simulink model "Quadrotor_eliminated_v2"  (R2020a)
settings: Solver=FixedStepAuto  StartTime=0.0  StopTime=options.T_train  FixedStep=options.dt  RelTol=1e-6
undefined symbols (not defined in the file or in its folder): options, Quad
libraries: neural x179, simulink x2
(part 3 of 10)

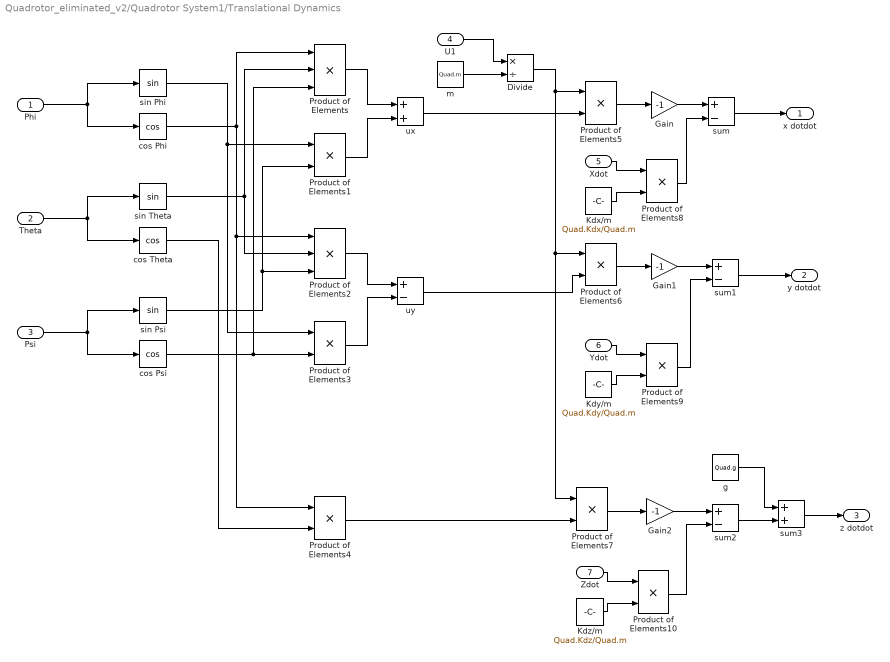
== system Quadrotor_eliminated_v2/Quadrotor System1/Translational Dynamics ==
  Phi : Inport
  Theta : Inport  Port=2
  Psi : Inport  Port=3
  U1 : Inport  Port=4
  Xdot : Inport  Port=5
  Ydot : Inport  Port=6
  Zdot : Inport  Port=7
  Divide : Product  Inputs=*/
  Gain : Gain  Gain=-1
  Gain1 : Gain  Gain=-1
  Gain2 : Gain  Gain=-1
  Kdx/m : Constant  Value=Quad.Kdx/Quad.m
  Kdy/m : Constant  Value=Quad.Kdy/Quad.m
  Kdz/m : Constant  Value=Quad.Kdz/Quad.m
  Product of Elements : Product  Inputs=3
  Product of Elements{1,3..10} (9 alike) : Product
  Product of Elements2 : Product  Inputs=3
  cos Phi : Trigonometry  Operator=cos
  cos Psi : Trigonometry  Operator=cos
  cos Theta : Trigonometry  Operator=cos
  g : Constant  Value=Quad.g
  m : Constant  Value=Quad.m
  sin Phi : Trigonometry
  sin Psi : Trigonometry
  sin Theta : Trigonometry
  sum : Sum  Inputs=+-
  sum1 : Sum  Inputs=+-
  sum2 : Sum  Inputs=+-
  sum3 : Sum
  ux : Sum
  uy : Sum  Inputs=+-
  x dotdot : Outport  VectorParamsAs1DForOutWhenUnconnected=off
  y dotdot : Outport  Port=2  VectorParamsAs1DForOutWhenUnconnected=off
  z dotdot : Outport  Port=3  VectorParamsAs1DForOutWhenUnconnected=off
  wires:
  Phi/1 -> sin Phi/1, cos Phi/1
  Theta/1 -> sin Theta/1, cos Theta/1
  Psi/1 -> sin Psi/1, cos Psi/1
  sin Theta/1 -> Product of Elements/2, Product of Elements2/2
  cos Psi/1 -> Product of Elements/3, Product of Elements3/2
  cos Phi/1 -> Product of Elements/1, Product of Elements2/1, Product of Elements4/1
  sin Phi/1 -> Product of Elements1/1, Product of Elements3/1
  sin Psi/1 -> Product of Elements1/2, Product of Elements2/3
  Product of Elements/1 -> ux/1
  Product of Elements1/1 -> ux/2
  ux/1 -> Product of Elements5/2
  Product of Elements2/1 -> uy/1
  Product of Elements3/1 -> uy/2
  uy/1 -> Product of Elements6/2
  cos Theta/1 -> Product of Elements4/2
  Product of Elements4/1 -> Product of Elements7/2
  U1/1 -> Divide/1
  m/1 -> Divide/2
  Divide/1 -> Product of Elements5/1, Product of Elements6/1, Product of Elements7/1
  sum3/1 -> z dotdot/1
  Product of Elements5/1 -> Gain/1
  Product of Elements6/1 -> Gain1/1
  Xdot/1 -> Product of Elements8/1
  Kdx/m/1 -> Product of Elements8/2
  Gain/1 -> sum/1
  Product of Elements8/1 -> sum/2
  sum/1 -> x dotdot/1
  Ydot/1 -> Product of Elements9/1
  Kdy/m/1 -> Product of Elements9/2
  Gain1/1 -> sum1/1
  Product of Elements9/1 -> sum1/2
  sum1/1 -> y dotdot/1
  Zdot/1 -> Product of Elements10/1
  Kdz/m/1 -> Product of Elements10/2
  Product of Elements7/1 -> Gain2/1
  g/1 -> sum3/1
  sum2/1 -> sum3/2
  Product of Elements10/1 -> sum2/2
  Gain2/1 -> sum2/1

== system Quadrotor_eliminated_v2/Quadrotor System2/Angular Velocities Transformation ==
  Theta : Inport
  Phi : Inport  Port=2
  Phi dot : Inport  Port=3
  Theta dot : Inport  Port=4
  Psi dot : Inport  Port=5
  Product : Product  RndMeth=Zero
  Product1 : Product  RndMeth=Zero
  Product2 : Product  Inputs=3  RndMeth=Zero
  Product3 : Product  RndMeth=Zero
  Product4 : Product  Inputs=3  RndMeth=Zero
  Sum : Sum  Inputs=+-
  Sum1 : Sum
  Sum2 : Sum
  sin : Trigonometry
  sin{1,4..6} (4 alike) : Trigonometry  Operator=cos
  sin2 : Trigonometry
  sin3 : Trigonometry
  p : Outport  VectorParamsAs1DForOutWhenUnconnected=off
  q : Outport  Port=2  VectorParamsAs1DForOutWhenUnconnected=off
  r : Outport  Port=3  VectorParamsAs1DForOutWhenUnconnected=off
  wires:
  Phi dot/1 -> Sum/1
  Theta/1 -> sin4/1, sin6/1, sin/1
  sin/1 -> Product/1
  Psi dot/1 -> Product/2, Product2/3, Product4/1
  Product/1 -> Sum/2
  Sum/1 -> p/1
  Phi/1 -> sin1/1, sin2/1, sin3/1, sin5/1
  sin1/1 -> Product1/1
  Theta dot/1 -> Product1/2, Product3/1
  Product1/1 -> Sum1/1
  sin2/1 -> Product2/1
  sin4/1 -> Product2/2
  Product2/1 -> Sum1/2
  Sum1/1 -> q/1
  sin3/1 -> Product3/2
  sin5/1 -> Product4/2
  sin6/1 -> Product4/3
  Product3/1 -> Sum2/1
  Product4/1 -> Sum2/2
  Sum2/1 -> r/1

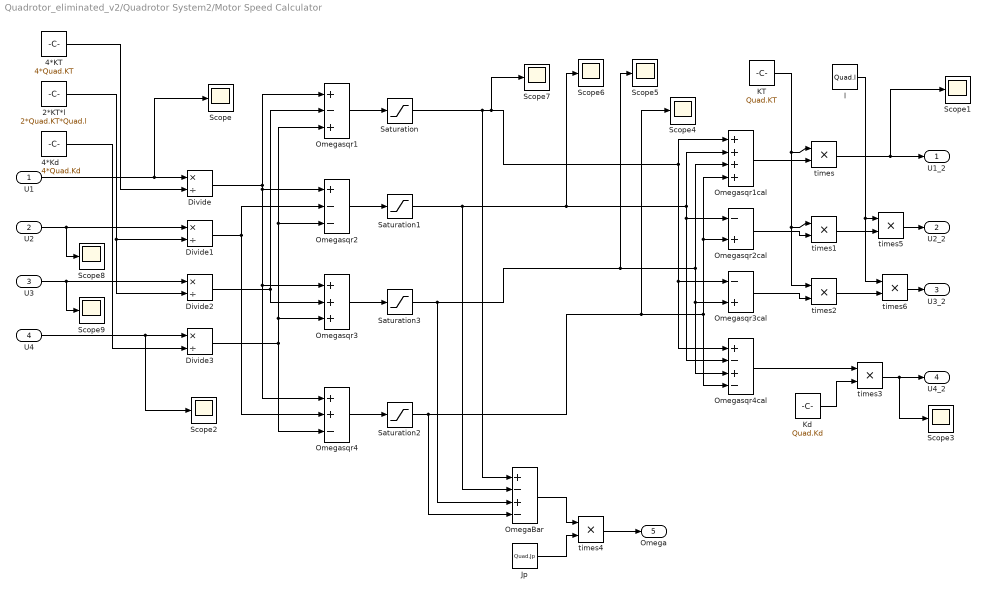
== system Quadrotor_eliminated_v2/Quadrotor System2/Motor Speed Calculator ==
  U1 : Inport
  U2 : Inport  Port=2
  U3 : Inport  Port=3
  U4 : Inport  Port=4
  2*KT*l : Constant  Value=2*Quad.KT*Quad.l
  4*KT : Constant  Value=4*Quad.KT
  4*Kd : Constant  Value=4*Quad.Kd
  Divide{,1..3} (4 alike) : Product  Inputs=*/
  Jp : Constant  Value=Quad.Jp
  KT : Constant  Value=Quad.KT
  Kd : Constant  Value=Quad.Kd
  OmegaBar : Sum  Inputs=+-+-
  Omegasqr1 : Sum  Inputs=+-+
  Omegasqr1cal : Sum  Inputs=++++
  Omegasqr2 : Sum  Inputs=+--
  Omegasqr2cal : Sum  Inputs=-+
  Omegasqr3 : Sum  Inputs=+++
  Omegasqr3cal : Sum  Inputs=-+
  Omegasqr4 : Sum  Inputs=++-
  Omegasqr4cal : Sum  Inputs=+-+-
  Saturation{,1..3} (4 alike) : Saturate  UpperLimit=Quad.max_motor_speed^2  LowerLimit=Quad.min_motor_speed^2  ZeroCross=off
  Scope{,1..9} (10 alike) : Scope
  l : Constant  Value=Quad.l
  times{,1..6} (7 alike) : Product  Inputs=**
  U1_2 : Outport  VectorParamsAs1DForOutWhenUnconnected=off
  U2_2 : Outport  Port=2  VectorParamsAs1DForOutWhenUnconnected=off
  U3_2 : Outport  Port=3  VectorParamsAs1DForOutWhenUnconnected=off
  U4_2 : Outport  Port=4  VectorParamsAs1DForOutWhenUnconnected=off
  Omega : Outport  Port=5  VectorParamsAs1DForOutWhenUnconnected=off
  wires:
  U1/1 -> Divide/1, Scope/1
  4*KT/1 -> Divide/2
  U2/1 -> Divide1/1, Scope8/1
  2*KT*l/1 -> Divide1/2, Divide2/2
  U3/1 -> Divide2/1, Scope9/1
  U4/1 -> Divide3/1, Scope2/1
  4*Kd/1 -> Divide3/2
  Divide/1 -> Omegasqr1/1, Omegasqr2/1, Omegasqr3/1, Omegasqr4/1
  Divide2/1 -> Omegasqr1/2, Omegasqr3/2
  Divide3/1 -> Omegasqr1/3, Omegasqr2/3, Omegasqr3/3, Omegasqr4/3
  Divide1/1 -> Omegasqr2/2, Omegasqr4/2
  OmegaBar/1 -> times4/1
  times4/1 -> Omega/1
  KT/1 -> times/1, times1/1, times2/1
  Omegasqr1cal/1 -> times/2
  Omegasqr2cal/1 -> times1/2
  Omegasqr3cal/1 -> times2/2
  Omegasqr4cal/1 -> times3/1
  Kd/1 -> times3/2
  times/1 -> U1_2/1, Scope1/1
  times3/1 -> U4_2/1, Scope3/1
  Jp/1 -> times4/2
  times5/1 -> U2_2/1
  times6/1 -> U3_2/1
  l/1 -> times5/1, times6/1
  times1/1 -> times5/2
  times2/1 -> times6/2
  Saturation/1 -> OmegaBar/1, Omegasqr1cal/1, Omegasqr3cal/1, Omegasqr4cal/1, Scope7/1
  Saturation2/1 -> OmegaBar/4, Omegasqr1cal/4, Omegasqr2cal/2, Omegasqr4cal/4, Scope4/1
  Saturation3/1 -> OmegaBar/3, Omegasqr1cal/3, Omegasqr3cal/2, Omegasqr4cal/3, Scope5/1
  Saturation1/1 -> OmegaBar/2, Omegasqr1cal/2, Omegasqr2cal/1, Omegasqr4cal/2, Scope6/1
  Omegasqr1/1 -> Saturation/1
  Omegasqr2/1 -> Saturation1/1
  Omegasqr3/1 -> Saturation3/1
  Omegasqr4/1 -> Saturation2/1

== system Quadrotor_eliminated_v2/Quadrotor System2/Rotational Dynamics ==
  p : Inport
  q : Inport  Port=2
  r : Inport  Port=3
  U2 : Inport  Port=4
  U3 : Inport  Port=5
  U4 : Inport  Port=6
  Omega : Inport  Port=7
  (Jx-Jy)/Jz : Constant  Value=(Quad.Jx - Quad.Jy)/Quad.Jz
  (Jy-Jz)/Jx : Constant  Value=(Quad.Jy - Quad.Jz)/Quad.Jx
  (Jz-Jx)/Jy : Constant  Value=(Quad.Jz - Quad.Jx)/Quad.Jy
  1/Jz : Constant  Value=1/Quad.Jz
  Add : Sum  Inputs=+-+
  Add1 : Sum  Inputs=+++
  Add2 : Sum
  Jp/Jx : Constant  Value=Quad.Jp/Quad.Jx
  Jp/Jy : Constant  Value=Quad.Jp/Quad.Jy
  Product of Elements{,1,3..4,6} (5 alike) : Product  Inputs=3
  Product of Elements2 : Product
  Product of Elements5 : Product
  Product of Elements7 : Product
  l/Jx : Constant  Value=Quad.l/Quad.Jx
  l/Jy : Constant  Value=Quad.l/Quad.Jy
  Phi dot dot : Outport  VectorParamsAs1DForOutWhenUnconnected=off
  Theta dot dot : Outport  Port=2  VectorParamsAs1DForOutWhenUnconnected=off
  Psi dot dot : Outport  Port=3  VectorParamsAs1DForOutWhenUnconnected=off
  wires:
  Product of Elements/1 -> Add/1
  Product of Elements1/1 -> Add/2
  Product of Elements2/1 -> Add/3
  Add/1 -> Phi dot dot/1
  (Jy-Jz)/Jx/1 -> Product of Elements/1
  q/1 -> Product of Elements/2, Product of Elements1/2, Product of Elements6/3
  r/1 -> Product of Elements/3, Product of Elements3/3
  Jp/Jx/1 -> Product of Elements1/1
  l/Jx/1 -> Product of Elements2/1
  U2/1 -> Product of Elements2/2
  Omega/1 -> Product of Elements1/3, Product of Elements4/3
  Product of Elements3/1 -> Add1/1
  Product of Elements4/1 -> Add1/2
  Product of Elements5/1 -> Add1/3
  Add1/1 -> Theta dot dot/1
  (Jz-Jx)/Jy/1 -> Product of Elements3/1
  Jp/Jy/1 -> Product of Elements4/1
  l/Jy/1 -> Product of Elements5/1
  U3/1 -> Product of Elements5/2
  p/1 -> Product of Elements3/2, Product of Elements4/2, Product of Elements6/2
  Product of Elements7/1 -> Add2/2
  Add2/1 -> Psi dot dot/1
  U4/1 -> Product of Elements7/2
  1/Jz/1 -> Product of Elements7/1
  (Jx-Jy)/Jz/1 -> Product of Elements6/1
  Product of Elements6/1 -> Add2/1

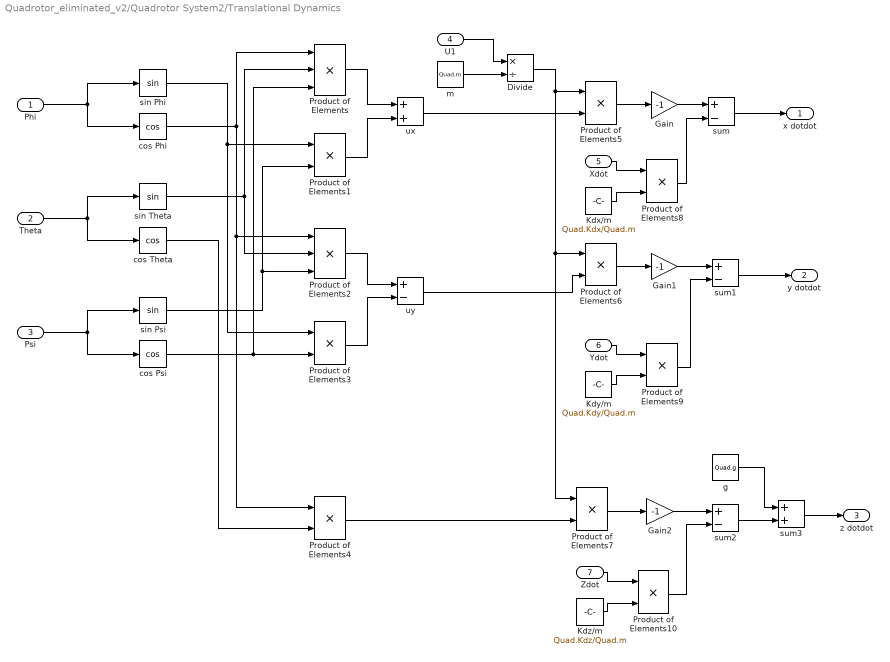
== system Quadrotor_eliminated_v2/Quadrotor System2/Translational Dynamics ==
  Phi : Inport
  Theta : Inport  Port=2
  Psi : Inport  Port=3
  U1 : Inport  Port=4
  Xdot : Inport  Port=5
  Ydot : Inport  Port=6
  Zdot : Inport  Port=7
  Divide : Product  Inputs=*/
  Gain : Gain  Gain=-1
  Gain1 : Gain  Gain=-1
  Gain2 : Gain  Gain=-1
  Kdx/m : Constant  Value=Quad.Kdx/Quad.m
  Kdy/m : Constant  Value=Quad.Kdy/Quad.m
  Kdz/m : Constant  Value=Quad.Kdz/Quad.m
  Product of Elements : Product  Inputs=3
  Product of Elements{1,3..10} (9 alike) : Product
  Product of Elements2 : Product  Inputs=3
  cos Phi : Trigonometry  Operator=cos
  cos Psi : Trigonometry  Operator=cos
  cos Theta : Trigonometry  Operator=cos
  g : Constant  Value=Quad.g
  m : Constant  Value=Quad.m
  sin Phi : Trigonometry
  sin Psi : Trigonometry
  sin Theta : Trigonometry
  sum : Sum  Inputs=+-
  sum1 : Sum  Inputs=+-
  sum2 : Sum  Inputs=+-
  sum3 : Sum
  ux : Sum
  uy : Sum  Inputs=+-
  x dotdot : Outport  VectorParamsAs1DForOutWhenUnconnected=off
  y dotdot : Outport  Port=2  VectorParamsAs1DForOutWhenUnconnected=off
  z dotdot : Outport  Port=3  VectorParamsAs1DForOutWhenUnconnected=off
  wires:
  Phi/1 -> sin Phi/1, cos Phi/1
  Theta/1 -> sin Theta/1, cos Theta/1
  Psi/1 -> sin Psi/1, cos Psi/1
  sin Theta/1 -> Product of Elements/2, Product of Elements2/2
  cos Psi/1 -> Product of Elements/3, Product of Elements3/2
  cos Phi/1 -> Product of Elements/1, Product of Elements2/1, Product of Elements4/1
  sin Phi/1 -> Product of Elements1/1, Product of Elements3/1
  sin Psi/1 -> Product of Elements1/2, Product of Elements2/3
  Product of Elements/1 -> ux/1
  Product of Elements1/1 -> ux/2
  ux/1 -> Product of Elements5/2
  Product of Elements2/1 -> uy/1
  Product of Elements3/1 -> uy/2
  uy/1 -> Product of Elements6/2
  cos Theta/1 -> Product of Elements4/2
  Product of Elements4/1 -> Product of Elements7/2
  U1/1 -> Divide/1
  m/1 -> Divide/2
  Divide/1 -> Product of Elements5/1, Product of Elements6/1, Product of Elements7/1
  sum3/1 -> z dotdot/1
  Product of Elements5/1 -> Gain/1
  Product of Elements6/1 -> Gain1/1
  Xdot/1 -> Product of Elements8/1
  Kdx/m/1 -> Product of Elements8/2
  Gain/1 -> sum/1
  Product of Elements8/1 -> sum/2
  sum/1 -> x dotdot/1
  Ydot/1 -> Product of Elements9/1
  Kdy/m/1 -> Product of Elements9/2
  Gain1/1 -> sum1/1
  Product of Elements9/1 -> sum1/2
  sum1/1 -> y dotdot/1
  Zdot/1 -> Product of Elements10/1
  Kdz/m/1 -> Product of Elements10/2
  Product of Elements7/1 -> Gain2/1
  g/1 -> sum3/1
  sum2/1 -> sum3/2
  Product of Elements10/1 -> sum2/2
  Gain2/1 -> sum2/1

== system Quadrotor_eliminated_v2/Translational Position PID Controller/Desired Position GF to BF ==
  X GF : Inport
  Y GF : Inport  Port=2
  Psi : Inport  Port=3
  Product{,1..3} (4 alike) : Product  RndMeth=Zero
  Sum : Sum
  Sum2 : Sum  Inputs=+-
  sin1 : Trigonometry  Operator=cos
  sin2 : Trigonometry
  "X Bf " : Outport  VectorParamsAs1DForOutWhenUnconnected=off
  Y Bf : Outport  Port=2  VectorParamsAs1DForOutWhenUnconnected=off
  wires:
  Psi/1 -> sin1/1, sin2/1
  sin1/1 -> Product/1, Product2/1
  X GF/1 -> Product/2, Product3/2
  Product/1 -> Sum/1
  sin2/1 -> Product1/1, Product3/1
  Y GF/1 -> Product1/2, Product2/2
  Product1/1 -> Sum/2
  Sum/1 -> "X Bf "/1
  Product2/1 -> Sum2/1
  Product3/1 -> Sum2/2
  Sum2/1 -> Y Bf/1

== system Quadrotor_eliminated_v2/Translational Position PID Controller/Position GF to BF ==
  X GF : Inport
  Y GF : Inport  Port=2
  Psi : Inport  Port=3
  Product{,1..3} (4 alike) : Product  RndMeth=Zero
  Sum : Sum
  Sum2 : Sum  Inputs=+-
  sin1 : Trigonometry  Operator=cos
  sin2 : Trigonometry
  "X Bf " : Outport  VectorParamsAs1DForOutWhenUnconnected=off
  Y Bf : Outport  Port=2  VectorParamsAs1DForOutWhenUnconnected=off
  wires:
  Psi/1 -> sin1/1, sin2/1
  sin1/1 -> Product/1, Product2/1
  X GF/1 -> Product/2, Product3/2
  Product/1 -> Sum/1
  sin2/1 -> Product1/1, Product3/1
  Y GF/1 -> Product1/2, Product2/2
  Product1/1 -> Sum/2
  Sum/1 -> "X Bf "/1
  Product2/1 -> Sum2/1
  Product3/1 -> Sum2/2
  Sum2/1 -> Y Bf/1

== system Quadrotor_eliminated_v2/Translational Position PID Controller/X PID ==
  X desired : Inport
  X : Inport  Port=2
  Derivative : Derivative
  Integrator : Integrator
  Kd : Gain  Gain=Quad.X_KD
  Ki : Gain  Gain=Quad.X_KI
  Kp : Gain  Gain=Quad.X_KP
  Saturation1 : Saturate  UpperLimit=Quad.theta_max  LowerLimit=-Quad.theta_max
  Saturation2 : Saturate  UpperLimit=Quad.theta_max  LowerLimit=-Quad.theta_max
  Sum : Sum  Inputs=---
  X Error : Sum  Inputs=+-
  Theta Desired : Outport  VectorParamsAs1DForOutWhenUnconnected=off
  wires:
  X/1 -> X Error/2, Derivative/1
  X desired/1 -> X Error/1
  Derivative/1 -> Kd/1
  Kp/1 -> Sum/1
  Sum/1 -> Saturation2/1
  X Error/1 -> Integrator/1, Kp/1
  Integrator/1 -> Ki/1
  Kd/1 -> Sum/3
  Saturation2/1 -> Theta Desired/1
  Ki/1 -> Saturation1/1
  Saturation1/1 -> Sum/2

== system Quadrotor_eliminated_v2/Translational Position PID Controller/Y PID ==
  Y desired : Inport
  Y : Inport  Port=2
  Derivative : Derivative
  Integrator : Integrator
  Kd : Gain  Gain=Quad.Y_KD
  Ki : Gain  Gain=Quad.Y_KI
  Kp : Gain  Gain=Quad.Y_KP
  Saturation1 : Saturate  UpperLimit=Quad.phi_max  LowerLimit=-Quad.phi_max
  Saturation2 : Saturate  UpperLimit=Quad.phi_max  LowerLimit=-Quad.phi_max
  Sum : Sum  Inputs=+++
  Y Error : Sum  Inputs=+-
  Phi Desired : Outport  VectorParamsAs1DForOutWhenUnconnected=off
  wires:
  Y/1 -> Y Error/2, Derivative/1
  Y desired/1 -> Y Error/1
  Derivative/1 -> Kd/1
  Kp/1 -> Sum/1
  Sum/1 -> Saturation2/1
  Y Error/1 -> Integrator/1, Kp/1
  Integrator/1 -> Ki/1
  Kd/1 -> Sum/3
  Ki/1 -> Saturation1/1
  Saturation1/1 -> Sum/2
  Saturation2/1 -> Phi Desired/1

== system Quadrotor_eliminated_v2/NN/Layer 1/Delays 1 ==
  "p{1}" : Inport  PortDimensions=15
      mask Display: e = 0.06;c1 = [120 230 180]/255;c2 = ([120 230 180]+0)/(256+128);c3 = ([120 230 180]+128)/(256+128);patch([0 1 1 0],[0 0 1 1],c1);patch([0 1 1 1-e 1-e 0+e],[0 0 1 1-e 0+e 0+e],c2);patch([0 0 1 1-e 0+e 0+e],[0 1 1 1-e 1-e 0+e],c3);plot([0 1 1 0 0],[0 0 1 1 0]);
  mux : Mux  Inputs=1
      mask Display: e = 0.06;c1 = [120 150 230]/255;c2 = ([120 150 230]+0)/383;c3 = ([120 150 230]+128)/383;patch([0 1 1 0],[0 0 1 1],c1);patch([0 1 1 1-e 1-e 0+e],[0 0 1 1-e 0+e 0+e],c2);patch([0 0 1 1-e 0+e 0+e],[0 1 1 1-e 1-e 0+e],c3);plot([0 1 1 0 0],[0 0 1 1 0]);disp('Mux')
  "pd{1,1}" : Outport
      mask Display: e = 0.06;c1 = [120 230 180]/255;c2 = ([120 230 180]+0)/(256+128);c3 = ([120 230 180]+128)/(256+128);patch([0 1 1 0],[0 0 1 1],c1);patch([0 1 1 1-e 1-e 0+e],[0 0 1 1-e 0+e 0+e],c2);patch([0 0 1 1-e 0+e 0+e],[0 1 1 1-e 1-e 0+e],c3);plot([0 1 1 0 0],[0 0 1 1 0]);
  wires:
  "p{1}"/1 -> mux/1
  mux/1 -> "pd{1,1}"/1
